simulink model "HDVSim_Hybrid_Truck_Platooning"  (R2018b)
settings: Solver=ode3  StartTime=0.0  StopTime=inf  FixedStep=sample_time  MaxStep=0.1  RelTol=1e-3  EnableMultiTasking=on
model workspace (MAT data in the model file):
  Anschaffungskosten = [3707764736; 2; 1; 1; 1; 1]
  Bat : struct (value not decoded)
  Driving_cycle = 18
  Eigenschaften = []
  Electric_Truck = 0
  Elektro_LKW = 0
  FuelCell : struct (value not decoded)
  Fueltype = 1
  Gewichte = [3707764736; 2; 1; 1; 2; 2]
  Hybrid_Truck = 0
  IZ12 = 3600
  Kraftstoff = 1
  M_el = 1000
  SOC_T_EM_completely_available = 0.5
  SOC_addition = 0.4
  SOC_el = 0.8
  SOC_target = 0.85
  Sailing_without_drag_torque = 0
  MCOS : class17 (value not decoded)
  TCO_Anhaenger = 1
  TCO_Trailer = 1
  T_distance_LPS_down = 250
  T_distance_LPS_up = 250
  VSim : struct (value not decoded)
  Vehicle = 'empty'
  WPT : struct (value not decoded)
  acquisition_costs = [3707764736; 2; 1; 1; 5; 5]
  addition_for_critical_slope = 0.01
  ambient : struct (value not decoded)
  auxiliary_consumers : struct (value not decoded)
  critical_altitude_difference = 50
  cycle : struct (value not decoded)
  dcycle = 18
  distance_1_PPC = 175
  distance_2_PPC = 200
  distance_PPC_altitude_difference = 10000
  driver : struct (value not decoded)
  em : struct (value not decoded)
  em_M_max = 1050
  engine : struct (value not decoded)
  final_drive : struct (value not decoded)
  ifElectric = 1
  ifOptimized = 0
  look_ahead_PPC = 250
  max_distance = 50000
  name = 'Verbrauchssimulation_Hybrid_LKW_Platooning'
  propertie = [3707764736; 2; 1; 1; 6; 6]
  prospective_cruise_control = 0
  sample_time = 0.1
  tank : struct (value not decoded)
  tires : struct (value not decoded)
  transmission : struct (value not decoded)
  v_PPC_delta = 2.77777777778
  v_max_electrical_drive_only = 13.8888888889
  vehicle : struct (value not decoded)
  vehicle_F_brake_max = 309890.14
  MCOS : class17 (value not decoded)
  x = 1
values from neighbouring files (symbols this model uses):
  transmission = Transmission_gearing(1, 1, false, false, final_drive.ratio)    [Parameterizing.m]
symbols that are objects in the model workspace (value not decoded): ambient, auxiliary_consumers, Bat, cycle, driver, em, engine, final_drive, tires, vehicle, WPT
undefined symbols (not defined in the file or in its folder): Ion, Lithium
libraries: simulink x23, powerlib x2, electricdrivelib x1
(part 2 of 3)

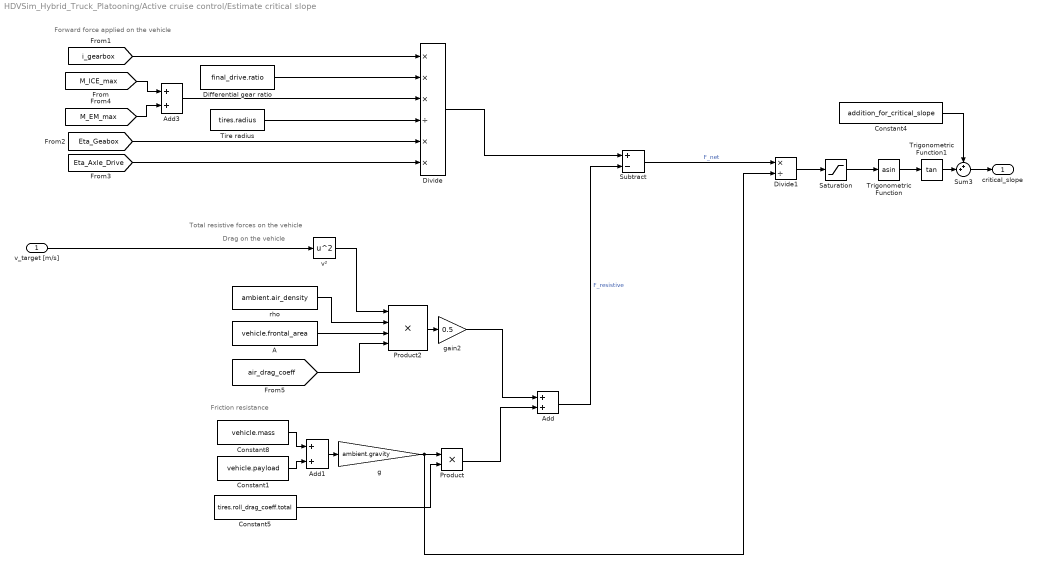
== system HDVSim_Hybrid_Truck_Platooning/Active cruise control/Estimate critical slope ==
  note: Total resistive forces on the vehicle
  note: Friction resistance
  note: Drag on the vehicle
  note: Forward force applied on the vehicle
  v_target [m/s] : Inport
  A : Constant  Value=vehicle.frontal_area
  Add : Sum
  Add1 : Sum
  Add3 : Sum
  Constant1 : Constant  Value=vehicle.payload
  Constant4 : Constant  Value=addition_for_critical_slope
  Constant5 : Constant  Value=tires.roll_drag_coeff.total
  Constant8 : Constant  Value=vehicle.mass
  Differential gear ratio : Constant  Value=final_drive.ratio
  Divide : Product  Inputs=***/**
  Divide1 : Product  Inputs=*/
  Product : Product
  Product2 : Product  Inputs=4  RndMeth=Zero
  Saturation : Saturate  UpperLimit=1  LowerLimit=-1
  Subtract : Sum  Inputs=+-
  Sum3 : Sum  Inputs=++|
  Tire radius : Constant  Value=tires.radius
  Trigonometric Function : Trigonometry  Operator=asin
  Trigonometric Function1 : Trigonometry  Operator=tan
  g : Gain  Gain=ambient.gravity
  gain2 : Gain  Gain=0.5
  rho : Constant  Value=ambient.air_density
  v² : Math  Operator=square  SaturateOnIntegerOverflow=on
  critical_slope : Outport
  wires:
  Add3/1 -> Divide/3
  [i_gearbox] -> Divide/1
  Differential gear ratio/1 -> Divide/2
  Tire radius/1 -> Divide/4
  Divide/1 -> Subtract/1
  Subtract/1 -> Divide1/1  "F_net"
  v²/1 -> Product2/1
  rho/1 -> Product2/2
  A/1 -> Product2/3
  [air_drag_coeff] -> Product2/4
  Product2/1 -> gain2/1
  Constant8/1 -> Add1/1
  Constant1/1 -> Add1/2
  Add1/1 -> g/1
  Constant5/1 -> Product/2
  Trigonometric Function/1 -> Trigonometric Function1/1
  Divide1/1 -> Saturation/1
  Sum3/1 -> critical_slope/1
  Constant4/1 -> Sum3/1
  Trigonometric Function1/1 -> Sum3/2
  v_target [m/s]/1 -> v²/1
  [Eta_Geabox] -> Divide/5
  [Eta_Axle_Drive] -> Divide/6
  [M_ICE_max] -> Add3/1
  [M_EM_max] -> Add3/2
  gain2/1 -> Add/1
  Product/1 -> Add/2
  Add/1 -> Subtract/2  "F_resistive"
  g/1 -> Product/1, Divide1/2
  Saturation/1 -> Trigonometric Function/1

== system HDVSim_Hybrid_Truck_Platooning/Driver controls/PI controller brake ==
  delta_v : Inport
  Add : Sum
  "I - controller " : Gain  Gain=driver.controller_integral_gain
  "Integrator, reset for sign change of delta v" : Integrator  ExternalReset=either  ZeroCross=off
  "P - controller " : Gain  Gain=driver.controller_proportional_gain
  F_target [N] : Outport
  wires:
  "Integrator, reset for sign change of delta v"/1 -> Add/2  "I_part"
  "I - controller "/1 -> "Integrator, reset for sign change of delta v"/1
  Add/1 -> F_target [N]/1  "F_target"
  "P - controller "/1 -> Add/1  "P_part"
  delta_v/1 -> "I - controller "/1, "Integrator, reset for sign change of delta v"/2, "P - controller "/1

== system HDVSim_Hybrid_Truck_Platooning/Driver controls/PI controller throttle1 ==
  delta_v : Inport
  Add : Sum
  "I - controller " : Gain  Gain=driver.controller_integral_gain
  "Integrator, reset for sign change of delta v" : Integrator  ExternalReset=either  ZeroCross=off
  "P - controller " : Gain  Gain=driver.controller_proportional_gain
  F_target [N] : Outport
  wires:
  "Integrator, reset for sign change of delta v"/1 -> Add/2  "I_part"
  "I - controller "/1 -> "Integrator, reset for sign change of delta v"/1
  Add/1 -> F_target [N]/1  "F_target"
  "P - controller "/1 -> Add/1  "P_partl"
  delta_v/1 -> "Integrator, reset for sign change of delta v"/2, "I - controller "/1, "P - controller "/1

== system HDVSim_Hybrid_Truck_Platooning/Driver controls/ZKU ==
  In1 : Inport
  Switch1 : Switch  Threshold=1
  zero1 : Constant  Value=0
  Out1 : Outport
  wires:
  zero1/1 -> Switch1/1
  [ZKU] -> Switch1/2
  Switch1/1 -> Out1/1
  In1/1 -> Switch1/3

== system HDVSim_Hybrid_Truck_Platooning/Driver controls/ZKU1 ==
  In1 : Inport
  Switch1 : Switch  Threshold=1
  zero1 : Constant  Value=0
  Out1 : Outport
  wires:
  In1/1 -> Switch1/3
  Switch1/1 -> Out1/1
  [ZKU] -> Switch1/2
  zero1/1 -> Switch1/1

== system HDVSim_Hybrid_Truck_Platooning/Driving cycle/Holding time at the beginning ==
  In1 : Inport
  Clock2 : Clock
  Constant3 : Constant  Value=cycle.stop_start
  Constant4 : Constant  Value=0
  Subtract1 : Sum  Inputs=+-
  Switch1 : Switch
  Out1 : Outport
  wires:
  In1/1 -> Switch1/1
  Constant3/1 -> Subtract1/2
  Clock2/1 -> Subtract1/1
  Constant4/1 -> Switch1/3
  Subtract1/1 -> Switch1/2
  Switch1/1 -> Out1/1

== system HDVSim_Hybrid_Truck_Platooning/Driving cycle/Holding time at the end ==
  In1 : Inport
  Clock1 : Clock
  Constant : Constant
  Constant1 : Constant  Value=cycle.stop_end
  Constant2 : Constant
  Hit Crossing : HitCross  HitCrossingDirection=rising
  Integrator : Integrator  ExternalReset=rising
  Subtract : Sum  Inputs=+-
  Sum1 : Sum  Inputs=|++
  Switch : Switch  Criteria=u2 > Threshold  Threshold=cycle.stop_end
  Out1 : Outport
  wires:
  In1/1 -> Integrator/2
  Constant/1 -> Integrator/1
  Subtract/1 -> Hit Crossing/1
  Integrator/1 -> Switch/1
  Hit Crossing/1 -> Out1/1
  Clock1/1 -> Switch/2
  Constant1/1 -> Sum1/2, Subtract/2
  Sum1/1 -> Switch/3
  Switch/1 -> Subtract/1
  Constant2/1 -> Sum1/1

== system HDVSim_Hybrid_Truck_Platooning/Driving cycle/Significant speed deviation ==
  In1 : Inport
  Clock : Clock
  Compare To Constant : simulink/Logic and Bit Operations/Compare To Constant  relop=>=  const=30  OutDataTypeStr=boolean
  Compare To Constant1 : simulink/Logic and Bit Operations/Compare To Constant  relop=>=  const=1000  OutDataTypeStr=boolean
  Compare To Constant2 : simulink/Logic and Bit Operations/Compare To Constant  relop=<=  const=0.1  OutDataTypeStr=boolean
  Compare To Constant3 : simulink/Logic and Bit Operations/Compare To Constant  relop=>=  const=1000  OutDataTypeStr=boolean
  Constant : Constant
  Constant1 : Constant  Value=0
  Constant2 : Constant
  Constant3 : Constant  Value=0
  Display : Display
  Display1 : Display
  Display2 : Display
  Gain : Gain  Gain=3.6
  Gain1 : Gain  Gain=3.6
  Integrator1 : Integrator  ExternalReset=either
  Integrator2 : Integrator  ExternalReset=either
  Logical Operator : Logic  Operator=OR  AllPortsSameDT=off  OutDataTypeStr=boolean
  Sum : Sum  Inputs=|+-
  Switch : Switch  Criteria=u2 > Threshold
  Switch1 : Switch  Criteria=u2 > Threshold
  stop_time : Lookup_n-D  NumberOfTableDimensions=1  BreakpointsForDimension1=cycle.distance  Table=cycle.stop_time  InterpMethod=Flat  RndMeth=Simplest  InputSameDT=on
  Out1 : Outport
  wires:
  In1/1 -> stop_time/1
  stop_time/1 -> Sum/2
  [delta_v] -> Gain/1
  [v_current2] -> Gain1/1
  Gain/1 -> Compare To Constant/1
  Integrator2/1 -> Display/1, Compare To Constant1/1
  Compare To Constant1/1 -> Logical Operator/2
  Gain1/1 -> Compare To Constant2/1
  Integrator1/1 -> Sum/1
  Sum/1 -> Display1/1, Compare To Constant3/1
  Compare To Constant3/1 -> Logical Operator/1
  Logical Operator/1 -> Out1/1
  Switch1/1 -> Integrator2/1, Integrator2/2
  Switch/1 -> Integrator1/2, Integrator1/1
  Constant/1 -> Switch/1
  Compare To Constant2/1 -> Switch/2
  Constant1/1 -> Switch/3
  Constant2/1 -> Switch1/1
  Compare To Constant/1 -> Switch1/2
  Constant3/1 -> Switch1/3
  Clock/1 -> Display2/1

== system HDVSim_Hybrid_Truck_Platooning/ECU/Approach to stop ==
  stop_time [s] : Inport
  Clock : Clock
  Compare To Constant1 : simulink/Logic and Bit Operations/Compare To Constant  relop=<=  const=3  OutDataTypeStr=boolean
  Compare To Zero : simulink/Logic and Bit Operations/Compare To Zero  relop=<=  OutDataTypeStr=boolean
  Constant : Constant
  Constant1 : Constant  Value=3.1
  Constant2 : Constant
  Hit Crossing : HitCross  HitCrossingDirection=rising
  Integrator : Integrator  ExternalReset=rising  InitialCondition=0.001
  Integrator1 : Integrator  ExternalReset=rising
  Subtract : Sum  Inputs=+-
  Switch : Switch  Criteria=u2 > Threshold  Threshold=3
  Driver_M : Outport
  Driver_B : Outport  Port=2
  wires:
  Constant/1 -> Integrator/1
  stop_time [s]/1 -> Integrator/2, Subtract/2
  Integrator/1 -> Subtract/1
  Subtract/1 -> Compare To Zero/1, Hit Crossing/1
  Constant2/1 -> Integrator1/1
  Hit Crossing/1 -> Integrator1/2
  Clock/1 -> Switch/2
  Constant1/1 -> Switch/3
  Integrator1/1 -> Switch/1
  Switch/1 -> Compare To Constant1/1
  Compare To Constant1/1 -> Driver_M/1
  Compare To Zero/1 -> Driver_B/1

== system HDVSim_Hybrid_Truck_Platooning/ECU/Ausrollversuch ==
  note: Zusatndsautomat, der nach vorgegebener Zeit nach Erreichen von 85 km/h die Steuersignale
      | für ICE und EM gleich null setzt, um den Lkw ausrollen zu lassen
      | % Wolff 2018
  U_EM : Inport
  U_ICE : Inport  Port=2
  Chart1 : Stateflow chart  TreatAsAtomicUnit=on
  Chart2 : Stateflow chart  TreatAsAtomicUnit=on
  Scope2 : Scope  NumInputPorts=2
  U_EM_out : Outport
  U_ICE_out : Outport  Port=2
  wires:
  U_EM/1 -> Chart2/1(In)
  U_ICE/1 -> Chart1/1(In)
  [v_current2] -> Chart1/2(v_current), Chart2/2(v_current)
  Chart2/1(Out) -> U_EM_out/1, Scope2/2
  Chart1/1(Out) -> U_ICE_out/1, Scope2/1

== system HDVSim_Hybrid_Truck_Platooning/ECU/Calculations for braking ==
  note: Breaking from motor's regenerative breaking
  note: Breaking from disk brakes
  M_EM_max [Nm] : Inport
  Driver_B : Inport  Port=2
  Gear : Inport  Port=3
  Differential efficiency : Constant  Value=final_drive.trq_eff
  Differential gear ratio : Constant  Value=final_drive.ratio
  Divide : Product  Inputs=*/
  Divide1 : Product  Inputs=**/*/
  Efficiencies : Lookup  InputValues=[1:length(transmission.ratios)]  Table=transmission.trq_eff  LookUpMeth=Use Input Nearest
  Gearing : Lookup  InputValues=[1:length(transmission.ratios)]  Table=transmission.ratios  LookUpMeth=Use Input Nearest
  Maximum breaking force [N] : Constant  Value=vehicle.F_brake_max
  Product : Product
  Tire radius : Constant  Value=tires.radius
  F_brake_required [N] : Outport
  F_brake_elec_max [N] : Outport  Port=2
  wires:
  M_EM_max [Nm]/1 -> Divide1/1
  Divide/1 -> F_brake_elec_max [N]/1
  Divide1/1 -> Divide/1
  Tire radius/1 -> Divide/2
  Driver_B/1 -> Product/1
  Maximum breaking force [N]/1 -> Product/2
  Product/1 -> F_brake_required [N]/1
  Gear/1 -> Efficiencies/1, Gearing/1
  Gearing/1 -> Divide1/2
  Efficiencies/1 -> Divide1/3
  Differential gear ratio/1 -> Divide1/4
  Differential efficiency/1 -> Divide1/5

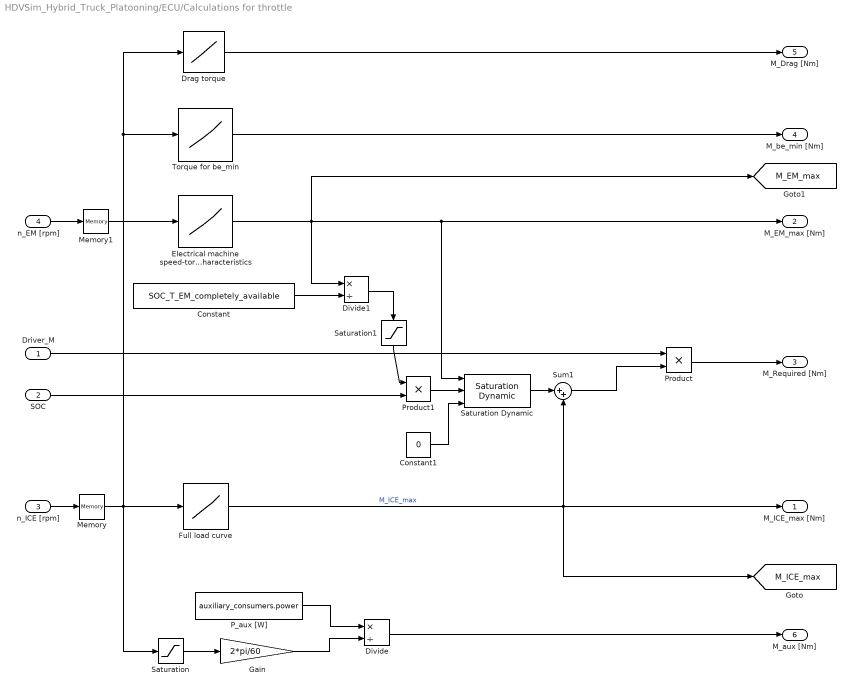
== system HDVSim_Hybrid_Truck_Platooning/ECU/Calculations for throttle ==
  Driver_M : Inport
  SOC : Inport  Port=2
  n_ICE [rpm] : Inport  Port=3
  n_EM [rpm] : Inport  Port=4
  Constant : Constant  Value=SOC_T_EM_completely_available
  Constant1 : Constant  Value=0
  Divide : Product  Inputs=*/
  Divide1 : Product  Inputs=*/
  Drag torque : Lookup  InputValues=engine.drag_torque.speed  Table=engine.drag_torque.trq  LookUpMeth=Interpolation-Use End Values
  Electrical machine speed-torque characteristics : Lookup_n-D  NumberOfTableDimensions=1  BreakpointsForDimension1=em.speed  Table=em.trq  ExtrapMethod=Clip  RndMeth=Simplest  InputSameDT=on
  Full load curve : Lookup  InputValues=engine.full_load.speed  Table=engine.full_load.trq  LookUpMeth=Interpolation-Use End Values
  Gain : Gain  Gain=2*pi/60
  Memory : Memory
  Memory1 : Memory
  P_aux [W] : Constant  Value=auxiliary_consumers.power
  Product : Product
  Product1 : Product
  Saturation : Saturate  UpperLimit=inf  LowerLimit=0.001
  Saturation Dynamic : simulink/Discontinuities/Saturation Dynamic  OutMin=[]  OutMax=[]  OutDataTypeStr=Inherit: Same as second input  OutDataType=fixdt(1, 16)  OutScaling=2^-10  DoSatur=off
  Saturation1 : Saturate  UpperLimit=1000000  LowerLimit=0.0000001
  Sum1 : Sum  Inputs=|++
  Torque for be_min : Lookup_n-D  NumberOfTableDimensions=1  BreakpointsForDimension1=engine.bsfc.speed  Table=engine.bsfc.M_be_min  ExtrapMethod=Clip  RndMeth=Simplest  InputSameDT=on
  M_ICE_max [Nm] : Outport
  M_EM_max [Nm] : Outport  Port=2
  M_Required [Nm] : Outport  Port=3
  M_be_min [Nm] : Outport  Port=4
  M_Drag [Nm] : Outport  Port=5
  M_aux [Nm] : Outport  Port=6
  tag scope: M_EM_max=global, M_ICE_max=global
  wires:
  Full load curve/1 -> [M_ICE_max], Sum1/2, M_ICE_max [Nm]/1  "M_ICE_max"
  Torque for be_min/1 -> M_be_min [Nm]/1
  Sum1/1 -> Product/2
  Product/1 -> M_Required [Nm]/1
  Drag torque/1 -> M_Drag [Nm]/1
  n_ICE [rpm]/1 -> Memory/1
  Gain/1 -> Divide/2
  P_aux [W]/1 -> Divide/1
  Divide/1 -> M_aux [Nm]/1
  Electrical machine speed-torque characteristics/1 -> Saturation Dynamic/1, M_EM_max [Nm]/1, [M_EM_max], Divide1/1
  Product1/1 -> Saturation Dynamic/2
  Saturation/1 -> Gain/1
  n_EM [rpm]/1 -> Memory1/1
  Memory/1 -> Saturation/1, Full load curve/1, Torque for be_min/1, Drag torque/1
  Memory1/1 -> Electrical machine speed-torque characteristics/1
  Constant/1 -> Divide1/2
  Saturation Dynamic/1 -> Sum1/1
  Constant1/1 -> Saturation Dynamic/3
  SOC/1 -> Product1/2
  Driver_M/1 -> Product/1
  Divide1/1 -> Saturation1/1
  Saturation1/1 -> Product1/1

== system HDVSim_Hybrid_Truck_Platooning/Electric motor/Machine current demand ==
  note: Electric power calculation
  "n_EM " : Inport
  M_EM_target [Nm] : Inport  Port=2
  Eff_EM : Inport  Port=3
  U_Bat [V] : Inport  Port=4
  Divide : Product  Inputs=*/*
  Divide1 : Product  Inputs=*/
  Gain : Gain  Gain=2*pi/60
  Saturation1 : Saturate  UpperLimit=inf  LowerLimit=1
  I_target [A] : Outport
  wires:
  Divide/1 -> Divide1/1
  Divide1/1 -> I_target [A]/1
  Gain/1 -> Divide/3
  M_EM_target [Nm]/1 -> Divide/1
  "n_EM "/1 -> Saturation1/1
  U_Bat [V]/1 -> Divide1/2
  Eff_EM/1 -> Divide/2
  Saturation1/1 -> Gain/1

== system HDVSim_Hybrid_Truck_Platooning/Electric motor/Machine torque demand ==
  n_EM [rpm] : Inport
  I_current [A] : Inport  Port=2
  Eff_EM : Inport  Port=3
  U_Bat [V] : Inport  Port=4
  Divide : Product  Inputs=*/*
  Gain : Gain  Gain=2*pi/60
  Product : Product
  Saturation1 : Saturate  UpperLimit=inf  LowerLimit=1
  M_EM [Nm] : Outport
  wires:
  U_Bat [V]/1 -> Product/1
  n_EM [rpm]/1 -> Saturation1/1
  Product/1 -> Divide/1
  Gain/1 -> Divide/2
  I_current [A]/1 -> Product/2
  Eff_EM/1 -> Divide/3
  Saturation1/1 -> Gain/1
  Divide/1 -> M_EM [Nm]/1

== system HDVSim_Hybrid_Truck_Platooning/ICE engine/Additional consumptions ==
  M_ICE_bfor_aux [Nm] : Inport
  n_clutch_en [rpm] : Inport  Port=2
  "1/min -> 1/s" : Gain  Gain=1/60
  2*pi : Constant  Value=2*pi
  Add : Sum
  Clock : Clock
  Constant : Constant  Value=0
  Constant1 : Constant  Value=Hybrid_Truck
  Gain : Gain  Gain=1000
  M_ICE_bfor_aux - M_aux [Nm] : Sum  Inputs=+-
  P_aux [W] : Constant  Value=auxiliary_consumers.power
  P_coolingSystem in kW : Lookup_n-D  NumberOfTableDimensions=1  BreakpointsSpecification=Even spacing  BreakpointsForDimension1=1:2400  Table=auxiliary_consumers.coolingSystem  ExtrapMethod=Clip  UseLastTableValue=on  InternalRulePriority=Speed  RndMeth=Simplest  InputSameDT=on
  Product1 : Product  Inputs=*//  RndMeth=Zero
  Scope : Scope
  Switch : Switch  Criteria=u2 ~= 0
  M_ICE_aftr_aux [Nm] : Outport
  wires:
  n_clutch_en [rpm]/1 -> "1/min -> 1/s"/1
  "1/min -> 1/s"/1 -> Product1/3
  2*pi/1 -> Product1/2
  P_aux [W]/1 -> Add/2
  Product1/1 -> Switch/3  "M_NV"
  M_ICE_bfor_aux [Nm]/1 -> M_ICE_bfor_aux - M_aux [Nm]/1
  M_ICE_bfor_aux - M_aux [Nm]/1 -> M_ICE_aftr_aux [Nm]/1
  Constant/1 -> Switch/1
  Switch/1 -> M_ICE_bfor_aux - M_aux [Nm]/2
  Constant1/1 -> Switch/2
  Clock/1 -> P_coolingSystem in kW/1
  P_coolingSystem in kW/1 -> Gain/1
  Add/1 -> Scope/1, Product1/1
  Gain/1 -> Add/1  "P_cs [W]"

== system HDVSim_Hybrid_Truck_Platooning/ICE engine/Consumption ==
  note: Amount of fuel calculation
  note: Fuel economy & emissions
  note: Fuel mass flow
  M [Nm] : Inport
  n [rpm] : Inport  Port=2
  CO2 emissions : Subsystem
  CO2 emissions g/t*km : Subsystem
  Compare To Constant : simulink/Logic and Bit Operations/Compare To Constant  relop=>=  const=0.3  OutDataTypeStr=uint8  ZeroCross=off
  Compare To Zero : simulink/Logic and Bit Operations/Compare To Zero  relop=<=  OutDataTypeStr=uint8  ZeroCross=off
  Constant : Constant  Value=0
  Engine torque-speed table : Lookup_n-D  BreakpointsForDimension1=engine.bsfc.trq  BreakpointsForDimension2=engine.bsfc.speed  BeginIndexSearchUsingPreviousIndexResult=on  Table=engine.bsfc.be  ExtrapMethod=Clip  UseLastTableValue=on  InternalRulePriority=Speed  RndMeth=Nearest
  Fuel economy Liter/100km : Subsystem
  Fuel economy Liter/t*km : Subsystem
  Idle consumption : Constant  Value=engine.idle_fuel_consumption
  Integrator : Integrator
  MinMax : MinMax  Function=max  Inputs=2  ZeroCross=off
  Product5 : Product  RndMeth=Zero
  Product8 : Product  RndMeth=Zero
  Saturation1 : Saturate  UpperLimit=engine.M_max  LowerLimit=0  ZeroCross=off
  Switch : Switch  Threshold=1  ZeroCross=off
  Terminator : Terminator
  Terminator1 : Terminator
  Terminator2 : Terminator
  g/h->l/h : Gain  Gain=1/engine.fuel.density
  "l/h -> l/s" : Gain  Gain=1/3600
  m->km : Gain  Gain=1/1000
  "n->omega, min->s" : Gain  Gain=pi/30000
  tag scope: Consumption_absolute_l=global, Consumption_l_per_100km=global
  wires:
  [s_current2] -> m->km/1
  Fuel economy Liter/100km/1(l/100km) -> [Consumption_l_per_100km]  "Fuel economy [l/100km]"
  CO2 emissions/1(g CO2/km) -> Terminator/1  "Fuel economy [gCO2/km]"
  m->km/1 -> Fuel economy Liter/100km/2(s [km]), CO2 emissions/2(s [km]), Fuel economy Liter/t*km/2(s [km]), CO2 emissions g/t*km/2(s [km]), Compare To Constant/1
  Fuel economy Liter/t*km/1(l/100t,km) -> Terminator1/1  "Fuel economy [l/100t.km]"
  Compare To Constant/1 -> Fuel economy Liter/100km/Enable, CO2 emissions g/t*km/Enable, Fuel economy Liter/t*km/Enable, CO2 emissions/Enable
  n [rpm]/1 -> Engine torque-speed table/2, Product5/2
  Product5/1 -> "n->omega, min->s"/1
  CO2 emissions g/t*km/1(g CO2/(t*km)) -> Terminator2/1  "Consumption [gCO2/(t.km)]"
  Product8/1 -> g/h->l/h/1  "g/h"
  Engine torque-speed table/1 -> Product8/1  "be[g/kWh]"
  "n->omega, min->s"/1 -> Product8/2
  g/h->l/h/1 -> MinMax/1
  Switch/1 -> "l/h -> l/s"/1  "fuel rate [l/h]"
  "l/h -> l/s"/1 -> Integrator/1
  Integrator/1 -> Fuel economy Liter/100km/1(B [l]), CO2 emissions/1(B [l]), Fuel economy Liter/t*km/1(B [l]), CO2 emissions g/t*km/1(B [l]), [Consumption_absolute_l]  "Volume [l]"
  Idle consumption/1 -> MinMax/2
  M [Nm]/1 -> Compare To Zero/1, Saturation1/1
  MinMax/1 -> Switch/3
  Constant/1 -> Switch/1
  Saturation1/1 -> Engine torque-speed table/1, Product5/1
  Compare To Zero/1 -> Switch/2

== system HDVSim_Hybrid_Truck_Platooning/ICE engine/maximum engine torque due to tire slip ==
  note: Overall transmission efficiency
  note: Wheel torque
  note: Wheel torque after losses & multiplications
  note: Overall transmission gear ratio
  Constant1 : Constant  Value=vehicle.Fx_max
  Differential efficiency : Constant  Value=final_drive.trq_eff
  Differential ratio : Constant  Value=final_drive.ratio
  Efficiencies : Lookup  InputValues=[1:length(transmission.ratios)]  Table=transmission.trq_eff  LookUpMeth=Use Input Nearest
  Gearing : Lookup  InputValues=[1:length(transmission.ratios)]  Table=transmission.ratios  LookUpMeth=Use Input Nearest
  Product : Product  Inputs=*//  RndMeth=Zero
  Product1 : Product  RndMeth=Zero
  Product2 : Product  Inputs=*//  RndMeth=Zero
  Tire radius : Constant  Value=tires.radius
  M_mot_max_traction [Nm] : Outport
  wires:
  Tire radius/1 -> Product1/2
  Constant1/1 -> Product1/1
  [gear] -> Efficiencies/1, Gearing/1
  Product1/1 -> Product/1  "M_rad_max_traction"
  Efficiencies/1 -> Product/2
  Gearing/1 -> Product/3
  Product/1 -> Product2/1
  Differential efficiency/1 -> Product2/2
  Differential ratio/1 -> Product2/3
  Product2/1 -> M_mot_max_traction [Nm]/1

== system HDVSim_Hybrid_Truck_Platooning/Power electronics & battery/Conversion of SOC ==
  SOC_absolut : Inport
  Constant : Constant  Value=0.5-Bat.Useable_range/2
  Constant1 : Constant  Value=0.5+Bat.Useable_range/2
  Divide : Product  Inputs=*/
  Saturation : Saturate  UpperLimit=1  LowerLimit=0
  Sum : Sum  Inputs=+-
  Sum1 : Sum  Inputs=-+
  SOC_relative : Outport
  wires:
  SOC_absolut/1 -> Sum/1
  Constant/1 -> Sum1/1, Sum/2
  Sum/1 -> Divide/1
  Constant1/1 -> Sum1/2
  Sum1/1 -> Divide/2
  Divide/1 -> Saturation/1
  Saturation/1 -> SOC_relative/1

== system HDVSim_Hybrid_Truck_Platooning/Power electronics & battery/Power electronics ==
  I_PE_current [A] : Inport
  1/Eta_LE : Gain  Gain=1/Bat.Efficiency_power_electronics
  Eta_LE : Gain  Gain=Bat.Efficiency_power_electronics
  Switch : Switch  Criteria=u2 > Threshold
  I_BAT_current [A] : Outport
  wires:
  Eta_LE/1 -> Switch/1
  1/Eta_LE/1 -> Switch/3
  I_PE_current [A]/1 -> 1/Eta_LE/1, Eta_LE/1, Switch/2
  Switch/1 -> I_BAT_current [A]/1

== system HDVSim_Hybrid_Truck_Platooning/Power electronics & battery/To prevent division by zero ==
  In1 : Inport
  In2 : Inport  Port=2
  In3 : Inport  Port=3
  Enable : EnablePort
  Abs : Abs
  Divide1 : Product  Inputs=*/
  Product1 : Product
  Out1 : Outport
  wires:
  In2/1 -> Product1/1
  In1/1 -> Product1/2
  In3/1 -> Divide1/1
  Product1/1 -> Divide1/2
  Divide1/1 -> Abs/1
  Abs/1 -> Out1/1  "Losses (%)"

== system HDVSim_Hybrid_Truck_Platooning/Summary/Subsystem ==
  E_DrivingResistance  in kWh : Inport
  E_System kWh : Inport  Port=2
  Enable : EnablePort
  Divide : Product  Inputs=*/
  eta_system : Outport
  wires:
  E_DrivingResistance  in kWh/1 -> Divide/1
  E_System kWh/1 -> Divide/2
  Divide/1 -> eta_system/1  "eta_system"

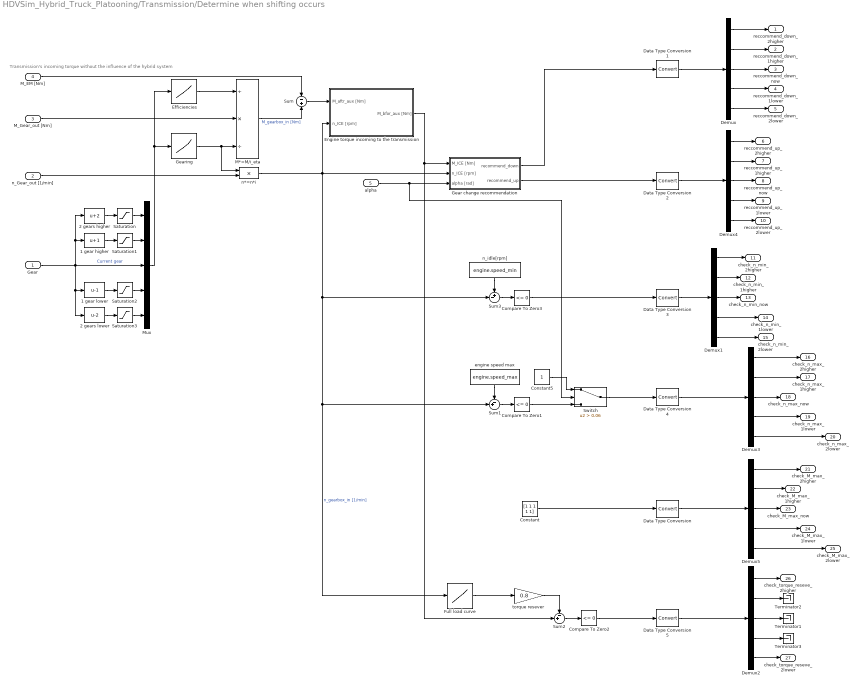
== system HDVSim_Hybrid_Truck_Platooning/Transmission/Determine when shifting occurs ==
  note: Transmission's incoming torque without the influence of the hybrid system
  Gear : Inport
  n_Gear_out [1/min] : Inport  Port=2
  M_Gear_out [Nm] : Inport  Port=3
  M_EM [Nm] : Inport  Port=4
  alpha : Inport  Port=5
  1 gear higher : Bias  Bias=1
  1 gear lower : Bias  Bias=-1
  2 gears higher : Bias  Bias=2
  2 gears lower : Bias  Bias=-2
  Compare To Zero1 : simulink/Logic and Bit Operations/Compare To Zero  relop=<=  OutDataTypeStr=boolean
  Compare To Zero2 : simulink/Logic and Bit Operations/Compare To Zero  relop=<=  OutDataTypeStr=boolean
  Compare To Zero3 : simulink/Logic and Bit Operations/Compare To Zero  relop=<=  OutDataTypeStr=boolean
  Constant : Constant  Value=[1 1 1 1 1]
  Constant5 : Constant
  Data Type Conversion{,1..5} (6 alike) : DataTypeConversion
  Demux{,1..5} (6 alike) : Demux  Outputs=5
  Efficiencies : Lookup  InputValues=[1:length(transmission.ratios)]  Table=transmission.trq_eff  LookUpMeth=Use Input Nearest
  Engine torque incoming to the transmission : Subsystem
  Full load curve : Lookup  InputValues=engine.full_load.speed  Table=engine.full_load.trq  LookUpMeth=Interpolation-Use End Values
  Gear change recommendation : Subsystem
  Gearing : Lookup  InputValues=[1:length(transmission.ratios)]  Table=transmission.ratios  LookUpMeth=Use Input Nearest
  M*=M/i_eta : Product  Inputs=/*/
  Mux : Mux  Inputs=5
  Saturation{,1..3} (4 alike) : Saturate  UpperLimit=length(transmission.ratios)  LowerLimit=0
  Sum : Sum  Inputs=-+
  Sum1 : Sum  Inputs=-+|
  Sum2 : Sum  Inputs=-+|
  Sum3 : Sum  Inputs=+-|
  Switch : Switch  Criteria=u2 > Threshold  Threshold=0.06
  Terminator1 : Terminator
  Terminator2 : Terminator
  Terminator3 : Terminator
  engine speed max : Constant  Value=engine.speed_max
  n*=n*i : Product  Inputs=**
  n_idle[rpm] : Constant  Value=engine.speed_min
  torque resever : Gain  Gain=0.8
  reccommend_down_2higher : Outport
  reccommend_down_1higher : Outport  Port=2
  reccommend_down_now : Outport  Port=3
  reccommend_down_1lower : Outport  Port=4
  reccommend_down_2lower : Outport  Port=5
  reccommend_up_2higher : Outport  Port=6
  reccommend_up_1higher : Outport  Port=7
  reccommend_up_now : Outport  Port=8
  reccommend_up_1lower : Outport  Port=9
  reccommend_up_2lower : Outport  Port=10
  check_n_min_2higher : Outport  Port=11
  check_n_min_1higher : Outport  Port=12
  check_n_min_now : Outport  Port=13
  check_n_min_1lower : Outport  Port=14
  check_n_min_2lower : Outport  Port=15
  check_n_max_2higher : Outport  Port=16
  check_n_max_1higher : Outport  Port=17
  check_n_max_now : Outport  Port=18
  check_n_max_1lower : Outport  Port=19
  check_n_max_2lower : Outport  Port=20
  check_M_max_2higher : Outport  Port=21
  check_M_max_1higher : Outport  Port=22
  check_M_max_now : Outport  Port=23
  check_M_max_1lower : Outport  Port=24
  check_M_max_2lower : Outport  Port=25
  check_torque_reseve_2higher : Outport  Port=26
  check_torque_reseve_2lower : Outport  Port=27
  wires:
  Gear/1 -> 1 gear lower/1, 2 gears lower/1, 1 gear higher/1, 2 gears higher/1, Mux/3  "Current gear"
  Engine torque incoming to the transmission/1(M_bfor_aux [Nm]) -> Sum2/2, Gear change recommendation/1(M_ICE [Nm])
  n*=n*i/1 -> Full load curve/1, Sum1/2, Sum3/2, Engine torque incoming to the transmission/2(n_ICE [rpm]), Gear change recommendation/2(n_ICE [rpm])  "n_gearbox_in [1/min]"
  n_Gear_out [1/min]/1 -> n*=n*i/2
  Efficiencies/1 -> M*=M/i_eta/1
  M_Gear_out [Nm]/1 -> M*=M/i_eta/2
  2 gears higher/1 -> Saturation/1
  1 gear higher/1 -> Saturation1/1
  Mux/1 -> Efficiencies/1, Gearing/1
  Demux/1 -> reccommend_down_2higher/1
  Demux/2 -> reccommend_down_1higher/1
  Demux/3 -> reccommend_down_now/1
  Demux2/1 -> check_torque_reseve_2higher/1
  Demux2/2 -> Terminator2/1
  Demux2/3 -> Terminator1/1
  Demux1/1 -> check_n_min_2higher/1
  Demux1/2 -> check_n_min_1higher/1
  Demux1/3 -> check_n_min_now/1
  Gearing/1 -> n*=n*i/1, M*=M/i_eta/3
  Saturation/1 -> Mux/1
  Saturation1/1 -> Mux/2
  1 gear lower/1 -> Saturation2/1
  Saturation2/1 -> Mux/4
  2 gears lower/1 -> Saturation3/1
  Saturation3/1 -> Mux/5
  Demux2/4 -> Terminator3/1
  Demux2/5 -> check_torque_reseve_2lower/1
  Demux/5 -> reccommend_down_2lower/1
  Demux/4 -> reccommend_down_1lower/1
  Demux1/4 -> check_n_min_1lower/1
  Demux1/5 -> check_n_min_2lower/1
  Demux4/1 -> reccommend_up_2higher/1
  Demux4/2 -> reccommend_up_1higher/1
  Demux4/3 -> reccommend_up_now/1
  Demux4/5 -> reccommend_up_2lower/1
  Demux4/4 -> reccommend_up_1lower/1
  Gear change recommendation/1(recommend_down) -> Data Type Conversion1/1
  Full load curve/1 -> torque resever/1
  torque resever/1 -> Sum2/1
  Sum2/1 -> Compare To Zero2/1
  Compare To Zero2/1 -> Data Type Conversion5/1
  Sum3/1 -> Compare To Zero3/1
  n_idle[rpm]/1 -> Sum3/1
  Gear change recommendation/2(recommend_up) -> Data Type Conversion2/1
  Demux3/1 -> check_n_max_2higher/1
  Demux3/2 -> check_n_max_1higher/1
  Demux3/3 -> check_n_max_now/1
  Demux3/4 -> check_n_max_1lower/1
  Demux3/5 -> check_n_max_2lower/1
  Sum1/1 -> Compare To Zero1/1
  engine speed max/1 -> Sum1/1
  Demux5/1 -> check_M_max_2higher/1
  Demux5/2 -> check_M_max_1higher/1
  Demux5/3 -> check_M_max_now/1
  Demux5/4 -> check_M_max_1lower/1
  Demux5/5 -> check_M_max_2lower/1
  Data Type Conversion1/1 -> Demux/1
  Data Type Conversion2/1 -> Demux4/1
  Data Type Conversion3/1 -> Demux1/1
  Data Type Conversion4/1 -> Demux3/1
  Data Type Conversion/1 -> Demux5/1
  Data Type Conversion5/1 -> Demux2/1
  Constant/1 -> Data Type Conversion/1
  Sum/1 -> Engine torque incoming to the transmission/1(M_aftr_aux [Nm])
  M*=M/i_eta/1 -> Sum/2  "M_gearbox_in [Nm]"
  M_EM [Nm]/1 -> Sum/1
  alpha/1 -> Switch/2, Gear change recommendation/3(alpha [rad])
  Compare To Zero1/1 -> Switch/3
  Switch/1 -> Data Type Conversion4/1
  Constant5/1 -> Switch/1
  Compare To Zero3/1 -> Data Type Conversion3/1

== system HDVSim_Hybrid_Truck_Platooning/Transmission/Torque flow through the transmission ==
  note: Outgoing torque from the transmission
  note: Rotational speed before and after the transmission
  M_gearbox_in [Nm] : Inport
  n_gearbox_out [1/min] : Inport  Port=2
  Gear : Inport  Port=3
  Divide : Product  Inputs=/
  Efficiencies : Lookup  InputValues=[1:length(transmission.ratios)]  Table=transmission.trq_eff  LookUpMeth=Use Input Nearest
  Gearing : Lookup  InputValues=[1:length(transmission.ratios)]  Table=transmission.ratios  LookUpMeth=Use Input Nearest
  M_Mot >= 0? : Switch  ZeroCross=off
  Product : Product  Inputs=***  RndMeth=Zero
  Rotating mass : Lookup  InputValues=[1:length(transmission.ratios)]  Table=transmission.lamda  LookUpMeth=Use Input Nearest
  n*=n*i : Product  Inputs=**
  n_gearbox_in [1/min] : Outport
  M_gearbox_out [Nm] : Outport  Port=2
  i_gearbox : Outport  Port=3
  tag scope: Eta_Geabox=global, lamda=global
  wires:
  Gearing/1 -> n*=n*i/1, i_gearbox/1, Product/3  "Gear ratio"
  n*=n*i/1 -> n_gearbox_in [1/min]/1
  Rotating mass/1 -> [lamda]  "lambda"
  n_gearbox_out [1/min]/1 -> n*=n*i/2
  Gear/1 -> Gearing/1, Rotating mass/1, Efficiencies/1
  M_gearbox_in [Nm]/1 -> M_Mot >= 0?/2, Product/2
  Product/1 -> M_gearbox_out [Nm]/1
  Efficiencies/1 -> Divide/1, M_Mot >= 0?/1  "Eta_Gearbox"
  Divide/1 -> M_Mot >= 0?/3
  M_Mot >= 0?/1 -> Product/1, [Eta_Geabox]

== system HDVSim_Hybrid_Truck_Platooning/Transmission/ZKU ==
  Gear : Inport
  Compare : simulink/Logic and Bit Operations/Compare To Zero  relop=>=  OutDataTypeStr=uint8  ZeroCross=off
  Constant : Constant  Value=-1
  Constant1 : Constant  Value=0
  Constant2 : Constant  Value=0
  Data Type Conversion : DataTypeConversion
  Derivative : Derivative
  Integrator : Integrator  ExternalReset=either  InitialCondition=transmission.shift_time
  Manual Switch : ManualSwitch
  Memory : Memory
  Switch : Switch  Threshold=1
  tag scope: ZKU=global
  wires:
  Constant/1 -> Integrator/1
  Derivative/1 -> Integrator/2
  Integrator/1 -> Compare/1
  Compare/1 -> Data Type Conversion/1
  Data Type Conversion/1 -> Switch/3
  Constant1/1 -> Manual Switch/2
  Gear/1 -> Manual Switch/1
  Manual Switch/1 -> Derivative/1
  [E_driving] -> Switch/2
  Constant2/1 -> Switch/1
  Switch/1 -> Memory/1
  Memory/1 -> [ZKU]

== system HDVSim_Hybrid_Truck_Platooning/Vehicle/Driving resistances without acceleration ==
  alpha [rad] : Inport
  v [m/s] : Inport  Port=2
  Add : Sum  Inputs=+++
  Drag : Subsystem
  Gradient resistance : Subsystem
  Rolling resistance : Subsystem
  F_W [N] : Outport
  tag scope: Air_drag=global, Rolling_drag=global
  wires:
  Drag/1(F_drag [N]) -> [Air_drag], Add/2
  Rolling resistance/1(F_Roll [N]) -> Add/1, [Rolling_drag]
  Add/1 -> F_W [N]/1
  v [m/s]/1 -> Drag/1(v [m/s])
  Gradient resistance/1(F_slope [N]) -> Add/3
  alpha [rad]/1 -> Gradient resistance/1(alpha [rad]), Rolling resistance/1(alpha [rad])

== system HDVSim_Hybrid_Truck_Platooning/Active cruise control/Estimate acceleration/Driving resistance without acceleration ==
  v [m/s] : Inport
  alpha [rad] : Inport  Port=2
  Add : Sum  Inputs=+++
  "Drag " : Subsystem
  Gradient resistance : Subsystem
  Rolling resistance : Subsystem
  F_x (resist) [N] : Outport
  wires:
  "Drag "/1(F_drag [N]) -> Add/2
  Rolling resistance/1(F_Roll [N]) -> Add/1
  Add/1 -> F_x (resist) [N]/1  "F_W"
  v [m/s]/1 -> "Drag "/1(v [m/s])
  Gradient resistance/1(F_slope [N]) -> Add/3
  alpha [rad]/1 -> Gradient resistance/1(alpha [rad]), Rolling resistance/1(alpha [rad])

== system HDVSim_Hybrid_Truck_Platooning/ICE engine/Consumption/CO2 emissions ==
  B [l] : Inport
  s [km] : Inport  Port=2
  Enable : EnablePort
  Divide : Product  Inputs=*/
  Product6 : Product  RndMeth=Zero
  "kg CO2 -> g CO2" : Gain  Gain=1000
  l->kg co2 : Constant  Value=engine.fuel.co2_per_litre
  g CO2/km : Outport
  wires:
  Product6/1 -> "kg CO2 -> g CO2"/1
  "kg CO2 -> g CO2"/1 -> Divide/1
  Divide/1 -> g CO2/km/1
  l->kg co2/1 -> Product6/1
  B [l]/1 -> Product6/2
  s [km]/1 -> Divide/2

== system HDVSim_Hybrid_Truck_Platooning/ICE engine/Consumption/CO2 emissions g//t*km ==
  B [l] : Inport
  s [km] : Inport  Port=2
  Enable : EnablePort
  Constant : Constant  Value=vehicle.payload
  g/tkm : Product  Inputs=*//
  kg CO2 : Product  RndMeth=Zero
  kg->g : Gain  Gain=1000
  l->kg co2 : Constant  Value=engine.fuel.co2_per_litre
  t->kg : Gain  Gain=1/1000
  g CO2/(t*km) : Outport
  wires:
  kg CO2/1 -> kg->g/1
  kg->g/1 -> g/tkm/1
  g/tkm/1 -> g CO2/(t*km)/1
  l->kg co2/1 -> kg CO2/1
  B [l]/1 -> kg CO2/2
  s [km]/1 -> g/tkm/2
  Constant/1 -> t->kg/1
  t->kg/1 -> g/tkm/3

== system HDVSim_Hybrid_Truck_Platooning/ICE engine/Consumption/Fuel economy Liter//100km ==
  B [l] : Inport
  s [km] : Inport  Port=2
  Enable : EnablePort
  Divide1 : Product  Inputs=*/
  l/km->l/100km : Gain  Gain=100
  l/100km : Outport
  wires:
  Divide1/1 -> l/km->l/100km/1
  l/km->l/100km/1 -> l/100km/1
  B [l]/1 -> Divide1/1
  s [km]/1 -> Divide1/2

== system HDVSim_Hybrid_Truck_Platooning/ICE engine/Consumption/Fuel economy Liter//t*km ==
  B [l] : Inport
  s [km] : Inport  Port=2
  Enable : EnablePort
  100km : Gain  Gain=100
  Constant : Constant  Value=vehicle.payload
  Divide1 : Product  Inputs=*//
  kg->t : Gain  Gain=1/1000
  l/100t,km : Outport
  wires:
  Divide1/1 -> l/100t,km/1
  B [l]/1 -> Divide1/1
  s [km]/1 -> 100km/1
  Constant/1 -> kg->t/1
  kg->t/1 -> Divide1/3
  100km/1 -> Divide1/2

== system HDVSim_Hybrid_Truck_Platooning/Transmission/Determine when shifting occurs/Engine torque incoming to the transmission ==
  note: Engine torque
  M_aftr_aux [Nm] : Inport
  n_ICE [rpm] : Inport  Port=2
  "1/min -> 1/s" : Gain  Gain=1/60
  2*pi : Constant  Value=2*pi
  Constant1 : Constant  Value=auxiliary_consumers.power
  M_ICE - M_aux : Sum
  Product1 : Product  Inputs=*//  RndMeth=Zero
  Saturation : Saturate  UpperLimit=inf  LowerLimit=0.001
  M_bfor_aux [Nm] : Outport
  wires:
  M_ICE - M_aux/1 -> M_bfor_aux [Nm]/1
  M_aftr_aux [Nm]/1 -> M_ICE - M_aux/1
  Product1/1 -> M_ICE - M_aux/2
  Constant1/1 -> Product1/1
  2*pi/1 -> Product1/2
  "1/min -> 1/s"/1 -> Product1/3
  n_ICE [rpm]/1 -> Saturation/1
  Saturation/1 -> "1/min -> 1/s"/1

== system HDVSim_Hybrid_Truck_Platooning/Transmission/Determine when shifting occurs/Gear change recommendation ==
  note: Gear change commands
  M_ICE [Nm] : Inport
  n_ICE [rpm] : Inport  Port=2
  alpha [rad] : Inport  Port=3
  Constant : Constant  Value=engine.shift_parameter.n1
  Constant1 : Constant  Value=engine.shift_parameter.n3
  Constant2 : Constant  Value=engine.shift_parameter.n2
  Constant3 : Constant  Value=engine.shift_parameter.n6
  Constant4 : Constant  Value=engine.shift_parameter.n5
  Constant5 : Constant  Value=0
  M_max [Nm] : Constant  Value=engine.shift_parameter.M_max
  Switch : Switch  Criteria=u2 > Threshold  Threshold=0.06
  recommend_down_calc_bsfc : Subsystem
  recommend_up_calc_bsfc : Subsystem
  recommend_down : Outport
  recommend_up : Outport  Port=2
  wires:
  M_max [Nm]/1 -> recommend_down_calc_bsfc/6(M_max [Nm]), recommend_up_calc_bsfc/6(M_max [Nm])  "M_max"
  n_ICE [rpm]/1 -> recommend_down_calc_bsfc/1(n), recommend_up_calc_bsfc/5(n)
  M_ICE [Nm]/1 -> recommend_up_calc_bsfc/1(M), recommend_down_calc_bsfc/2(M)
  recommend_down_calc_bsfc/1(Out1) -> recommend_down/1
  Constant/1 -> recommend_down_calc_bsfc/3(n_1)
  Constant1/1 -> recommend_down_calc_bsfc/4(n_3)
  Constant2/1 -> recommend_up_calc_bsfc/3(n_2), recommend_down_calc_bsfc/5(n_2)
  Constant3/1 -> recommend_up_calc_bsfc/2(n_6)
  Constant4/1 -> recommend_up_calc_bsfc/4(n_5)
  Constant5/1 -> Switch/1
  alpha [rad]/1 -> Switch/2
  recommend_up_calc_bsfc/1(recommend_up) -> Switch/3
  Switch/1 -> recommend_up/1

== system HDVSim_Hybrid_Truck_Platooning/Vehicle/Driving resistances without acceleration/Drag ==
  note: F_Drag = 0.5 * V^2 * rho * A * c_d
  note: Platooning Teil; Änderung c_w üder delta_x
  v [m/s] : Inport
  2-D Lookup Table : Lookup_n-D  BreakpointsSpecification=Even spacing  BreakpointsForDimension1=vehicle.cD_Data.d_T12  BreakpointsForDimension2=vehicle.cD_Data.d_T23  BreakpointsForDimension1FirstPoint=5  BreakpointsForDimension2FirstPoint=5  BreakpointsForDimension1Spacing=5  BreakpointsForDimension2Spacing=5  IndexSearchMethod=Evenly spaced points  Table=vehicle.air_drag_coeff  InternalRulePriority=Speed  RndMeth=Simplest  InputSameDT=on
  A : Constant  Value=vehicle.frontal_area
  Constant1 : Constant  Value=Driving_cycle
  Constant2 : Constant  Value=17
  Constant3 : Constant  Value=18
  Constant4 : Constant  Value=19
  Display : Display
  Logical Operator : Logic  Operator=OR  Inputs=3  AllPortsSameDT=off  OutDataTypeStr=boolean
  Mux : Mux  Inputs=2
  Product2 : Product  Inputs=4  RndMeth=Zero
  Relational Operator : RelationalOperator  Operator===  OutDataTypeStr=boolean  RndMeth=Simplest
  Relational Operator1 : RelationalOperator  Operator===  OutDataTypeStr=boolean  RndMeth=Simplest
  Relational Operator2 : RelationalOperator  Operator===  OutDataTypeStr=boolean  RndMeth=Simplest
  Scope : Scope  NumInputPorts=2
  Switch : Switch  Criteria=u2 > Threshold
  c_W : Constant  Value=vehicle.air_drag_coeff(end,end)
  gain2 : Gain  Gain=0.5
  rho : Constant  Value=ambient.air_density
  v² : Math  Operator=square  SaturateOnIntegerOverflow=on
  F_drag [N] : Outport
  tag scope: air_drag_coeff=global
  wires:
  v²/1 -> Product2/1
  gain2/1 -> F_drag [N]/1
  v [m/s]/1 -> v²/1
  rho/1 -> Product2/2
  A/1 -> Product2/3
  Product2/1 -> gain2/1
  2-D Lookup Table/1 -> Switch/1
  Logical Operator/1 -> Switch/2, Display/1
  Relational Operator1/1 -> Logical Operator/2
  Relational Operator2/1 -> Logical Operator/3
  Relational Operator/1 -> Logical Operator/1
  Constant2/1 -> Relational Operator/2
  Constant4/1 -> Relational Operator2/2
  c_W/1 -> Switch/3
  Switch/1 -> [air_drag_coeff], Scope/1, Product2/4  "c_D"
  Constant1/1 -> Relational Operator2/1, Relational Operator1/1, Relational Operator/1
  Constant3/1 -> Relational Operator1/2
  [delta_12] -> Mux/1, 2-D Lookup Table/1  "delta_T12"
  [delta_23] -> Mux/2, 2-D Lookup Table/2  "delta_T23"
  Mux/1 -> Scope/2  "Distance betw. Trucks"

== system HDVSim_Hybrid_Truck_Platooning/Vehicle/Driving resistances without acceleration/Gradient resistance ==
  note: F_slope = (m_tot * g) * sin(alpha)
  alpha [rad] : Inport
  Add : Sum
  Cargo weight : Constant  Value=vehicle.payload
  Product7 : Product  RndMeth=Zero
  Trigonometric Function : Trigonometry
  Vehicle weight : Constant  Value=vehicle.mass
  g : Gain  Gain=ambient.gravity
  F_slope [N] : Outport
  wires:
  alpha [rad]/1 -> Trigonometric Function/1
  Trigonometric Function/1 -> Product7/2
  Product7/1 -> F_slope [N]/1
  g/1 -> Product7/1
  Vehicle weight/1 -> Add/1
  Cargo weight/1 -> Add/2
  Add/1 -> g/1  "m_tot"

== system HDVSim_Hybrid_Truck_Platooning/Vehicle/Driving resistances without acceleration/Rolling resistance ==
  note: F_Roll = (m_tot * g) * mu * cos(alpha)
  alpha [rad] : Inport
  Add1 : Sum
  Cargo weight : Constant  Value=vehicle.payload
  Product7 : Product  Inputs=3  RndMeth=Zero
  Rolling friction coefficient : Constant  Value=tires.roll_drag_coeff.total
  Trigonometric Function : Trigonometry  Operator=cos
  Vehicle weight : Constant  Value=vehicle.mass
  g : Gain  Gain=ambient.gravity
  F_Roll [N] : Outport
  wires:
  alpha [rad]/1 -> Trigonometric Function/1
  Product7/1 -> F_Roll [N]/1
  Rolling friction coefficient/1 -> Product7/3  "mu"
  Trigonometric Function/1 -> Product7/1
  g/1 -> Product7/2
  Vehicle weight/1 -> Add1/1
  Cargo weight/1 -> Add1/2
  Add1/1 -> g/1  "m_tot"

== system HDVSim_Hybrid_Truck_Platooning/Active cruise control/Estimate acceleration/Driving resistance without acceleration/Drag  ==
  note: F_Drag = 0.5 * V^2 * rho * A * c_d
  v [m/s] : Inport
  A : Constant  Value=vehicle.frontal_area
  Product2 : Product  Inputs=4  RndMeth=Zero
  gain2 : Gain  Gain=0.5
  rho : Constant  Value=ambient.air_density
  v² : Math  Operator=square  SaturateOnIntegerOverflow=on
  F_drag [N] : Outport
  wires:
  v²/1 -> Product2/1
  gain2/1 -> F_drag [N]/1
  v [m/s]/1 -> v²/1
  rho/1 -> Product2/2
  A/1 -> Product2/3
  Product2/1 -> gain2/1
  [air_drag_coeff] -> Product2/4

== system HDVSim_Hybrid_Truck_Platooning/Active cruise control/Estimate acceleration/Driving resistance without acceleration/Gradient resistance ==
  note: F_slope = (m_tot * g) * sin(alpha)
  alpha [rad] : Inport
  Add : Sum
  Constant1 : Constant  Value=vehicle.payload
  Constant2 : Constant  Value=vehicle.mass
  Product7 : Product  RndMeth=Zero
  Trigonometric Function : Trigonometry
  g : Gain  Gain=ambient.gravity
  F_slope [N] : Outport
  wires:
  alpha [rad]/1 -> Trigonometric Function/1
  Trigonometric Function/1 -> Product7/2
  Product7/1 -> F_slope [N]/1
  g/1 -> Product7/1
  Constant2/1 -> Add/1
  Constant1/1 -> Add/2
  Add/1 -> g/1

== system HDVSim_Hybrid_Truck_Platooning/Active cruise control/Estimate acceleration/Driving resistance without acceleration/Rolling resistance ==
  note: F_Roll = (m_tot * g) * mu * cos(alpha)
  alpha [rad] : Inport
  Add1 : Sum
  Constant1 : Constant  Value=vehicle.payload
  Constant5 : Constant  Value=tires.roll_drag_coeff.total
  Constant8 : Constant  Value=vehicle.mass
  Product7 : Product  Inputs=3  RndMeth=Zero
  Trigonometric Function : Trigonometry  Operator=cos
  g : Gain  Gain=ambient.gravity
  F_Roll [N] : Outport
  wires:
  alpha [rad]/1 -> Trigonometric Function/1
  Product7/1 -> F_Roll [N]/1
  Constant5/1 -> Product7/3
  Trigonometric Function/1 -> Product7/1
  g/1 -> Product7/2
  Constant8/1 -> Add1/1
  Constant1/1 -> Add1/2
  Add1/1 -> g/1

== system HDVSim_Hybrid_Truck_Platooning/Transmission/Determine when shifting occurs/Gear change recommendation/recommend_down_calc_bsfc ==
  n : Inport
  M : Inport  Port=2
  n_1 : Inport  Port=3
  n_3 : Inport  Port=4
  n_2 : Inport  Port=5
  M_max [Nm] : Inport  Port=6
  Compare To Zero2 : simulink/Logic and Bit Operations/Compare To Zero  relop=<=  OutDataTypeStr=boolean
  Compare To Zero3 : simulink/Logic and Bit Operations/Compare To Zero  relop=<=  OutDataTypeStr=boolean
  MATLAB Function : MATLAB Function  TreatAsAtomicUnit=on
  Sum1 : Sum  Inputs=+-|
  Sum2 : Sum  Inputs=-+|
  logic2 : Logic  Operator=OR  AllPortsSameDT=off  OutDataTypeStr=boolean
  Out1 : Outport
  wires:
  n_1/1 -> MATLAB Function/3(n_1)  "n_1"
  n_3/1 -> MATLAB Function/4(n_3)
  Sum2/1 -> Compare To Zero2/1
  Sum1/1 -> Compare To Zero3/1
  MATLAB Function/1(g_1) -> Sum2/2
  Compare To Zero3/1 -> logic2/2
  logic2/1 -> Out1/1
  n/1 -> MATLAB Function/1(n), Sum1/1
  n_2/1 -> Sum1/2
  M/1 -> Sum2/1
  M_max [Nm]/1 -> MATLAB Function/2(M_max)
  Compare To Zero2/1 -> logic2/1

== system HDVSim_Hybrid_Truck_Platooning/Transmission/Determine when shifting occurs/Gear change recommendation/recommend_up_calc_bsfc ==
  M : Inport
  n_6 : Inport  Port=2
  n_2 : Inport  Port=3
  n_5 : Inport  Port=4
  n : Inport  Port=5
  M_max [Nm] : Inport  Port=6
  Compare To Zero : simulink/Logic and Bit Operations/Compare To Zero  relop=<=  OutDataTypeStr=boolean
  Compare To Zero1 : simulink/Logic and Bit Operations/Compare To Zero  relop=<=  OutDataTypeStr=boolean
  MATLAB Function1 : MATLAB Function  TreatAsAtomicUnit=on
  Sum1 : Sum  Inputs=-+|
  Sum2 : Sum  Inputs=+-|
  logic : Logic  AllPortsSameDT=off  OutDataTypeStr=boolean
  recommend_up : Outport
  wires:
  n_6/1 -> MATLAB Function1/3(n_6)
  Compare To Zero/1 -> logic/1
  logic/1 -> recommend_up/1
  n/1 -> Sum1/1, MATLAB Function1/1(n)
  n_2/1 -> MATLAB Function1/4(n_2)
  M_max [Nm]/1 -> MATLAB Function1/2(M_max)
  M/1 -> Sum2/1
  Sum2/1 -> Compare To Zero/1
  MATLAB Function1/1(g_2) -> Sum2/2
  n_5/1 -> Sum1/2
  Sum1/1 -> Compare To Zero1/1
  Compare To Zero1/1 -> logic/2
